simulink model "Discrete_Analog_Modelling"  (R2021b)
settings: Solver=VariableStepAuto  StartTime=0.0  StopTime=10.0  RelTol=1e-3
libraries: simulink_extras x1, simulink x1
settings Model: Creator=randy  LastModifiedBy=randy

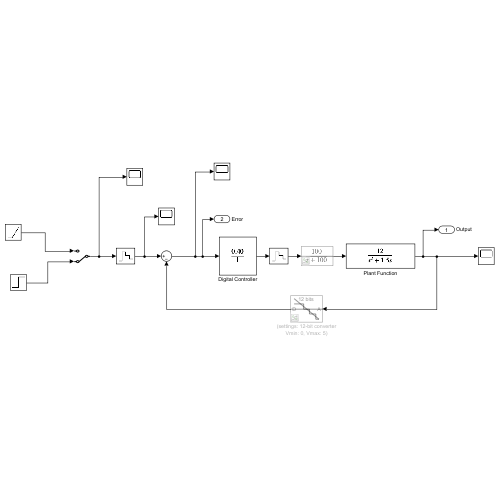
[thumbnail: Simulink's stored preview of the top-level diagram]
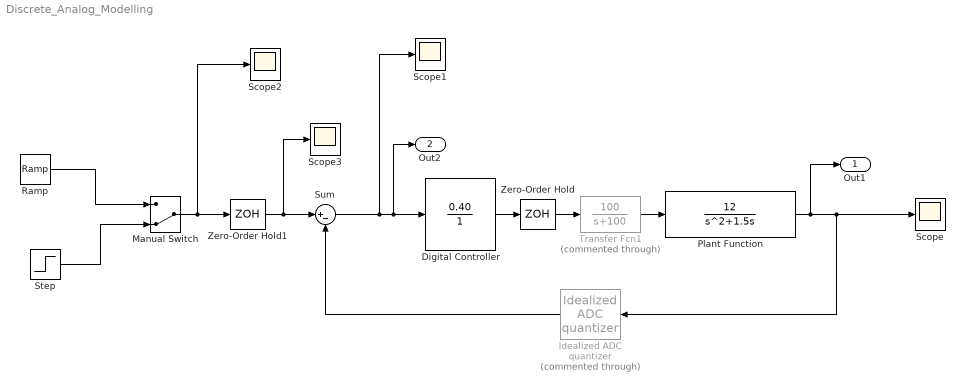
== system Discrete_Analog_Modelling ==
  Digital Controller : DiscreteTransferFcn  Numerator=[0.40]  Denominator=[1]  SampleTime=0.05
  Idealized ADC quantizer : simulink_extras/Additional Discrete/Idealized ADC quantizer  Commented=through  NumberOfConverterBits=12  Vmin=0  Vmax=5  OutputDataType=int16  OutputNegativeValues=off
  Manual Switch : ManualSwitch  CurrentSetting=0
  Plant Function : TransferFcn  Numerator=[12]  Denominator=[1 1.5 0 ]
  Ramp : simulink/Sources/Ramp  slope=1  start=0  InitialOutput=0
  Scope{,1..3} (4 alike) : Scope
  Step : Step  After=58  SampleTime=0
  Sum : Sum  Inputs=|+-
  Transfer Fcn1 : TransferFcn  Commented=through  Numerator=[100 ]  Denominator=[1 100]
  Zero-Order Hold : ZeroOrderHold  SampleTime=0.05
  Zero-Order Hold1 : ZeroOrderHold  SampleTime=0.05
  Out1 : Outport  SignalName=Output
  Out2 : Outport  Port=2  SignalName=Error
  wires:
  Transfer Fcn1/1 -> Plant Function/1
  Sum/1 -> Digital Controller/1, Out2/1, Scope1/1
  Zero-Order Hold/1 -> Transfer Fcn1/1
  Manual Switch/1 -> Zero-Order Hold1/1, Scope2/1
  Plant Function/1 -> Idealized ADC quantizer/1, Scope/1, Out1/1
  Digital Controller/1 -> Zero-Order Hold/1
  Ramp/1 -> Manual Switch/1
  Step/1 -> Manual Switch/2
  Idealized ADC quantizer/1 -> Sum/2
  Zero-Order Hold1/1 -> Scope3/1, Sum/1
